simulink model "draft_imu"  (R2023a)
settings: Solver=VariableStepAuto  StartTime=0.0  StopTime=10.0  RelTol=1e-3
values from neighbouring files (symbols this model uses):
  invTI0 = transpose(TI0)    [AttitudePlot.m]    (also in AttitudePlot_V0.m = T; Boomerang_4Wings.m; Boomerang_4Wings_Titan.m; Boomerang_4Wings_Venus52.m)
  omega = sim.omega    [Boomerang_4Wings.m]    (also in IMU_input.mat = [0 0.0801917548715 0.157805666526 0.231525909681 0.301269354)
  phi = phi1    [AttitudePlot.m]    (also in Boomerang_4Wings.m = sim.EulAng(:,1); Boomerang_4Wings_Titan.m = sim.EulAng(:,1); Boomerang_4Wings_Venus52.m = sim.EulAng(:,1); Boomerang_4Wings_Venus60.m = sim.EulAng(:,1))
  psi = psi1    [AttitudePlot.m]    (also in Boomerang_4Wings.m = sim.EulAng(:,3); Boomerang_4Wings_Titan.m = sim.EulAng(:,3); Boomerang_4Wings_Venus52.m = sim.EulAng(:,3); Boomerang_4Wings_Venus60.m = sim.EulAng(:,3))
  R_pos0 = [0; 0; 1.5]    [Boomerang_4Wings.m]    (also in Boomerang_4Wings_Titan.m; Boomerang_4Wings_Venus52.m; Boomerang_4Wings_Venus60.m; Boomerang_Cropped_Validation.m = [0; 0; 1.8])
  theta = theta1    [AttitudePlot.m]    (also in Boomerang_4Wings.m = sim.EulAng(:,2); Boomerang_4Wings_Titan.m = sim.EulAng(:,2); Boomerang_4Wings_Venus52.m = sim.EulAng(:,2); Boomerang_4Wings_Venus60.m = sim.EulAng(:,2))
  u0 = TI0*U0    [Boomerang_4Wings.m]    (also in Boomerang_4Wings_Titan.m; Boomerang_4Wings_Venus52.m; Boomerang_4Wings_Venus60.m; Boomerang_Cropped_Validation.m)
  udot = [3.69260558501 -4.82230918672 109.652400543 3.92433986557 -4.59965974133 116.960330022 3.85204924395 -4.67482269594 116.549650337 3.75753014323 -4.76891947229 115.561294646 ... (74205 elements, 3x24735)]    [IMU_input.mat]
libraries: aerolibnav x1
settings Model: Creator=dsantis  LastModifiedBy=dsantis

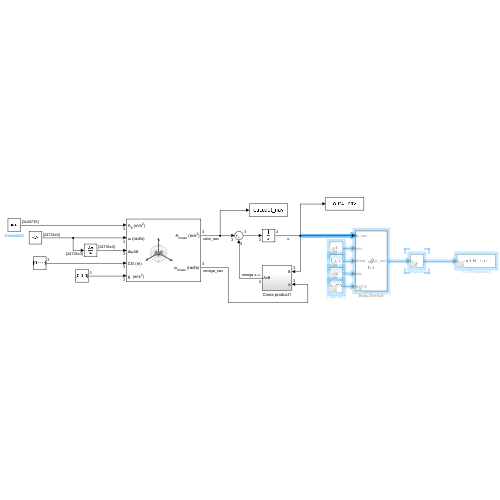
[thumbnail: Simulink's stored preview of the top-level diagram]
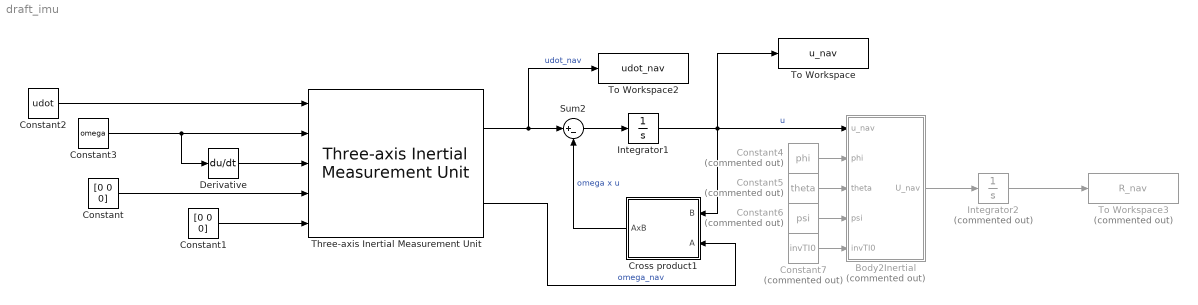
== system draft_imu ==
  Body2Inertial : MATLAB Function  Commented=on  TreatAsAtomicUnit=on
  Constant : Constant  Value=[0 0 0]
  Constant1 : Constant  Value=[0 0 0]
  Constant2 : Constant  Value=udot
  Constant3 : Constant  Value=omega
  Constant4 : Constant  Commented=on  Value=phi
  Constant5 : Constant  Commented=on  Value=theta
  Constant6 : Constant  Commented=on  Value=psi
  Constant7 : Constant  Commented=on  Value=invTI0
  Cross product1 : Subsystem
  Derivative : Derivative
  Integrator1 : Integrator  InitialCondition=u0
  Integrator2 : Integrator  Commented=on  InitialCondition=R_pos0
  Sum2 : Sum  Inputs=|+-
  Three-axis Inertial Measurement Unit : aerolibnav/Three-axis Inertial Measurement Unit  units=Metric (MKS)  imu=[0 0 0]  i_Ts=0  dtype_a=off  w_a=190  z_a=0.707  a_sf_cc=[1 0 0; 0 1 0; 0 0 1]  a_bias=[0 0 0]  a_sat="[-inf  -inf  -inf  inf inf inf]"  dtype_g=off  w_g=190  z_g=0.707  g_sf_cc=[1 0 0; 0 1 0; 0 0 1]  g_bias=[0 0 0]  g_sens=[0 0 0]  g_sat="[-inf  -inf  -inf  inf inf inf]"  i_rand=on  i_seeds=[23093 23094 23095 23096 23097 23098]  i_pow=[0.001 0.001 0.001 0.0001 0.0001 0.0001]
  To Workspace : ToWorkspace  VariableName=u_nav  SampleTime=-1
  To Workspace2 : ToWorkspace  VariableName=udot_nav  SampleTime=-1
  To Workspace3 : ToWorkspace  Commented=on  VariableName=R_nav  SampleTime=-1
  wires:
  Cross product1/1(AxB) -> Sum2/2  "omega x u"
  Three-axis Inertial Measurement Unit/2 -> Cross product1/2(A)  "omega_nav"
  Sum2/1 -> Integrator1/1
  Integrator1/1 -> Body2Inertial/1(u_nav), Cross product1/1(B), To Workspace/1  "u"
  Three-axis Inertial Measurement Unit/1 -> Sum2/1, To Workspace2/1  "udot_nav"
  Constant1/1 -> Three-axis Inertial Measurement Unit/5
  Derivative/1 -> Three-axis Inertial Measurement Unit/3
  Constant/1 -> Three-axis Inertial Measurement Unit/4
  Constant3/1 -> Derivative/1, Three-axis Inertial Measurement Unit/2
  Integrator2/1 -> To Workspace3/1
  Body2Inertial/1(U_nav) -> Integrator2/1
  Constant2/1 -> Three-axis Inertial Measurement Unit/1
  Constant4/1 -> Body2Inertial/2(phi)
  Constant5/1 -> Body2Inertial/3(theta)
  Constant6/1 -> Body2Inertial/4(psi)
  Constant7/1 -> Body2Inertial/5(invTI0)

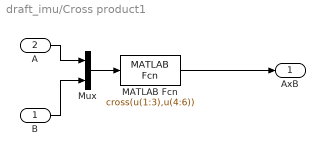
== system draft_imu/Cross product1 ==
  B : Inport
  A : Inport  Port=2
  MATLAB Fcn : MATLABFcn  MATLABFcn=cross(u(1:3),u(4:6))
  Mux : Mux  Inputs=2
  AxB : Outport  VectorParamsAs1DForOutWhenUnconnected=off
  wires:
  A/1 -> Mux/1
  B/1 -> Mux/2
  Mux/1 -> MATLAB Fcn/1
  MATLAB Fcn/1 -> AxB/1

== matlab function draft_imu/Body2Inertial ==
  data: u_nav input; phi input; theta input; psi input; invTI0 input; U_nav output
function U_nav  = fcn(u_nav, phi, theta, psi, invTI0)

R01 = [
    1, 0, 0;
    0, cos(phi), sin(phi);
    0, -sin(phi), cos(phi)
    ];
R02 = [
    cos(theta), 0, -sin(theta);
    0, 1, 0;
    sin(theta), 0, cos(theta)
];
R03 = [
    cos(psi), sin(psi), 0;
    -sin(psi), cos(psi), 0;
    0, 0, 1
];
T0 = R01*R02*R03;
invT0 = transpose(T0);

U_nav = invTI0*invT0*u_nav;
